simulink model "Grading_System"  (R2021a)
settings: Solver=FixedStepDiscrete  StartTime=0.0  StopTime=10.0  RelTol=1e-3
settings Model: Creator=Moamen_Hamed  LastModifiedBy=Moamen_Hamed
settings OptimizationCC: DefaultParameterBehavior=Inlined  EnhancedBackFolding=on  PassReuseOutputArgsAs=Individual arguments  OptimizeBlockOrder=speed  DifferentSizesBufferReuse=on  OptimizationCustomize=off  EfficientTunableParamExpr=on
settings DebuggingCC: ParameterTunabilityLossMsg=error
settings SFSimCC: MATLABDynamicMemAlloc=off
settings RTWCC: SystemTargetFile=ert.tlc  GenCodeOnly=on  TemplateMakefile=ert_default_tmf  GenerateReport=on  IncludeHyperlinkInReport=on  LaunchReport=on  GenerateTraceInfo=on
settings CodeAppCC: ForceParamTrailComments=on  IgnoreCustomStorageClasses=off  OperatorAnnotations=on  SimulinkDataObjDesc=on  SFDataObjDesc=on  InsertBlockDesc=on
settings ERTTargetCC: TargetLangStandard=C99 (ISO)  GenerateSampleERTMain=on  CodeInterfacePackaging=Reusable function  SupportComplex=off  InlinedParameterPlacement=NonHierarchical  ERTCustomFileTemplate=example_file_process.tlc

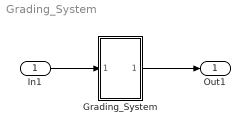
== system Grading_System ==
  In1 : Inport
  Grading_System : Subsystem  TreatAsAtomicUnit=on
  Out1 : Outport
  wires:
  In1/1 -> Grading_System/1(In1)
  Grading_System/1(Out1) -> Out1/1

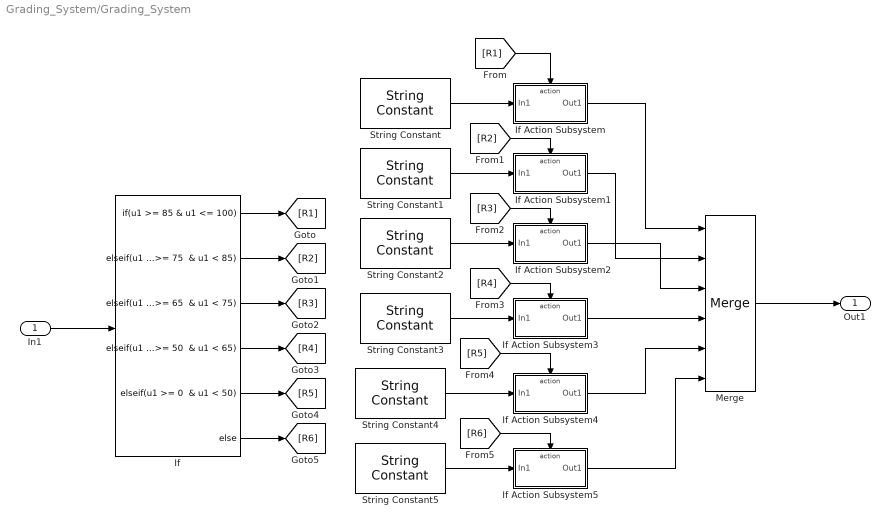
== system Grading_System/Grading_System ==
  In1 : Inport
  If : If  IfExpression=u1 >= 85 & u1 <= 100  ElseIfExpressions="u1 >= 75  & u1 < 85, u1 >= 65  & u1 < 75, u1 >= 50  & u1 < 65, u1 >= 0  & u1 < 50"
  If Action Subsystem : Subsystem  TreatAsAtomicUnit=on
  If Action Subsystem1 : Subsystem  TreatAsAtomicUnit=on
  If Action Subsystem2 : Subsystem  TreatAsAtomicUnit=on
  If Action Subsystem3 : Subsystem  TreatAsAtomicUnit=on
  If Action Subsystem4 : Subsystem  TreatAsAtomicUnit=on
  If Action Subsystem5 : Subsystem  TreatAsAtomicUnit=on
  Merge : Merge  Inputs=6
  String Constant : StringConstant  String="\"Excellent!\""
  String Constant1 : StringConstant  String="\"Very Good!\""
  String Constant2 : StringConstant  String="\"Good!\""
  String Constant3 : StringConstant  String="\"Pass!\""
  String Constant4 : StringConstant  String="\"Failed!\""
  String Constant5 : StringConstant  String="\"Invalid Input!\""
  Out1 : Outport
  wires:
  If/6 -> [R6]
  If/3 -> [R3]
  If Action Subsystem2/1(Out1) -> Merge/3
  [R2] -> If Action Subsystem1/Action
  If/2 -> [R2]
  If Action Subsystem/1(Out1) -> Merge/1
  String Constant2/1 -> If Action Subsystem2/1(In1)
  String Constant/1 -> If Action Subsystem/1(In1)
  [R4] -> If Action Subsystem3/Action
  String Constant1/1 -> If Action Subsystem1/1(In1)
  If/1 -> [R1]
  If Action Subsystem1/1(Out1) -> Merge/2
  If Action Subsystem4/1(Out1) -> Merge/5
  String Constant4/1 -> If Action Subsystem4/1(In1)
  If Action Subsystem5/1(Out1) -> Merge/6
  String Constant3/1 -> If Action Subsystem3/1(In1)
  If/4 -> [R4]
  String Constant5/1 -> If Action Subsystem5/1(In1)
  If/5 -> [R5]
  [R3] -> If Action Subsystem2/Action
  [R1] -> If Action Subsystem/Action
  If Action Subsystem3/1(Out1) -> Merge/4
  [R5] -> If Action Subsystem4/Action
  [R6] -> If Action Subsystem5/Action
  Merge/1 -> Out1/1
  In1/1 -> If/1

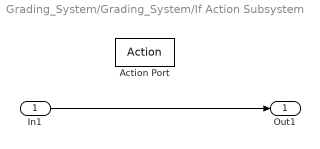
== system Grading_System/Grading_System/If Action Subsystem ==
  In1 : Inport
  Action Port : ActionPort  ActionPortLabel=if(u1 >= 85 & u1 <= 100)
  Out1 : Outport
  wires:
  In1/1 -> Out1/1

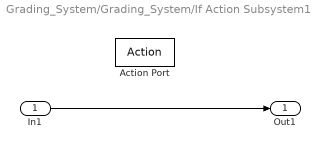
== system Grading_System/Grading_System/If Action Subsystem1 ==
  In1 : Inport
  Action Port : ActionPort  ActionPortLabel="elseif(u1 >= 75  & u1 < 85)"
  Out1 : Outport
  wires:
  In1/1 -> Out1/1

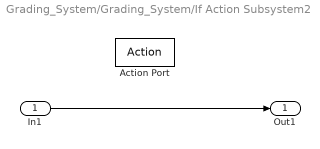
== system Grading_System/Grading_System/If Action Subsystem2 ==
  In1 : Inport
  Action Port : ActionPort  ActionPortLabel="elseif( u1 >= 65  & u1 < 75)"
  Out1 : Outport
  wires:
  In1/1 -> Out1/1

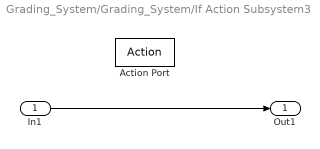
== system Grading_System/Grading_System/If Action Subsystem3 ==
  In1 : Inport
  Action Port : ActionPort  ActionPortLabel="elseif( u1 >= 50  & u1 < 65)"
  Out1 : Outport
  wires:
  In1/1 -> Out1/1

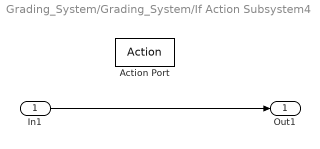
== system Grading_System/Grading_System/If Action Subsystem4 ==
  In1 : Inport
  Action Port : ActionPort  ActionPortLabel="elseif( u1 >= 0  & u1 < 50)"
  Out1 : Outport
  wires:
  In1/1 -> Out1/1

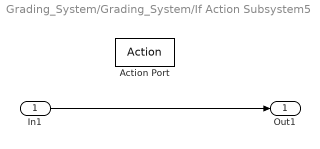
== system Grading_System/Grading_System/If Action Subsystem5 ==
  In1 : Inport
  Action Port : ActionPort  ActionPortLabel=else
  Out1 : Outport
  wires:
  In1/1 -> Out1/1
